simulink model "MIL_ASW"  (R2019b)
settings: Solver=FixedStepDiscrete  StartTime=0.0  StopTime=2  FixedStep=0.001  RelTol=1e-3  EnableMultiTasking=on
model workspace (MAT data in the model file):
  AccPedlCanVal : Simulink.Signal (value not decoded)
  AccPedlVal : Simulink.Signal (value not decoded)
  BrkPedlCanVal : Simulink.Signal (value not decoded)
  BrkPedlVal : Simulink.Signal (value not decoded)
  Cal1 : Simulink.Parameter (value not decoded)
  Cal10 : Simulink.Parameter (value not decoded)
  Cal11 : Simulink.Parameter (value not decoded)
  Cal12 : Simulink.Parameter (value not decoded)
  Cal2 : Simulink.Parameter (value not decoded)
  Cal3 : Simulink.Parameter (value not decoded)
  Cal4 : Simulink.Parameter (value not decoded)
  Cal5 : Simulink.Parameter (value not decoded)
  Cal6 : Simulink.Parameter (value not decoded)
  Cal7 : Simulink.Parameter (value not decoded)
  Cal8 : Simulink.Parameter (value not decoded)
  Cal9 : Simulink.Parameter (value not decoded)
  Clu1Act : Simulink.Signal (value not decoded)
  Clu1PTar : Simulink.Signal (value not decoded)
  Clu1Req : Simulink.Signal (value not decoded)
  Clu1TqTar : Simulink.Signal (value not decoded)
  Clu2Act : Simulink.Signal (value not decoded)
  Clu2PTar : Simulink.Signal (value not decoded)
  Clu2Req : Simulink.Signal (value not decoded)
  Clu2TqTar : Simulink.Signal (value not decoded)
  CluKissPtPLnch : Simulink.Parameter (value not decoded)
  CluOilTRawVal : Simulink.Signal (value not decoded)
  CluOilTVal : Simulink.Signal (value not decoded)
  CluOpenTqRatMax : Simulink.Parameter (value not decoded)
  CluPMap : Simulink.Parameter (value not decoded)
  CluPMax : Simulink.Parameter (value not decoded)
  CluPMaxGear1 : Simulink.Parameter (value not decoded)
  CluPMaxGear2 : Simulink.Parameter (value not decoded)
  CluPMaxGear3 : Simulink.Parameter (value not decoded)
  CluPMaxGear4 : Simulink.Parameter (value not decoded)
  CluPMaxGear5 : Simulink.Parameter (value not decoded)
  CluPMaxGear6 : Simulink.Parameter (value not decoded)
  CluPMaxGearR : Simulink.Parameter (value not decoded)
  CluPMin : Simulink.Parameter (value not decoded)
  CluPosnMax : Simulink.Parameter (value not decoded)
  CluSoln1IRawVal : Simulink.Signal (value not decoded)
  CluSoln1IReq : Simulink.Signal (value not decoded)
  CluSoln1IReqFlg : Simulink.Signal (value not decoded)
  CluSoln1IVal : Simulink.Signal (value not decoded)
  CluSoln1LineI : Simulink.Parameter (value not decoded)
  CluSoln1LineP : Simulink.Parameter (value not decoded)
  CluSoln1Pwm : Simulink.Signal (value not decoded)
  CluSoln2IRawVal : Simulink.Signal (value not decoded)
  CluSoln2IReq : Simulink.Signal (value not decoded)
  CluSoln2IReqFlg : Simulink.Signal (value not decoded)
  CluSoln2IVal : Simulink.Signal (value not decoded)
  CluSoln2LineI : Simulink.Parameter (value not decoded)
  CluSoln2LineP : Simulink.Parameter (value not decoded)
  CluSoln2Pwm : Simulink.Signal (value not decoded)
  CluTqMap : Simulink.Parameter (value not decoded)
  CrnkSpdRawVal : Simulink.Signal (value not decoded)
  CrnkSpdVal : Simulink.Signal (value not decoded)
  Drive_Intensity_Fuzzy : object (value not decoded)
  DrvIntenFzzy : Simulink.LookupTable (value not decoded)
  EngNIdle : Simulink.Parameter (value not decoded)
  EngNIdleMin : Simulink.Parameter (value not decoded)
  EngSpdCanVal : Simulink.Signal (value not decoded)
  EngThrCanVal : Simulink.Signal (value not decoded)
  EngTqAdd : Simulink.Parameter (value not decoded)
  EngTqCanVal : Simulink.Signal (value not decoded)
  EngTqIntvFlg : Simulink.Signal (value not decoded)
  EngTqIntvRat : Simulink.Signal (value not decoded)
  EngTqMapExtChartc : Simulink.Parameter (value not decoded)
  EngTqMapSpdIndx : Simulink.Parameter (value not decoded)
  EngTqMapThrtIndx : Simulink.Parameter (value not decoded)
  EngTqMapTqMax : Simulink.Parameter (value not decoded)
  EngTqMaxNorm : Simulink.Parameter (value not decoded)
  EngTqRef : Simulink.Parameter (value not decoded)
  EvenCluPRawVal : Simulink.Signal (value not decoded)
  EvenCluPVal : Simulink.Signal (value not decoded)
  EvenInpSpdRawVal : Simulink.Signal (value not decoded)
  EvenInpSpdVal : Simulink.Signal (value not decoded)
  FcnCallTime : Simulink.Parameter (value not decoded)
  FinalRat : Simulink.Parameter (value not decoded)
  Fork1A : Simulink.Parameter (value not decoded)
  Fork1Act : Simulink.Signal (value not decoded)
  Fork1B : Simulink.Parameter (value not decoded)
  Fork1DeltaSpdTar : Simulink.Parameter (value not decoded)
  Fork1MaxSpd1A : Simulink.Parameter (value not decoded)
  Fork1MaxSpd1B : Simulink.Parameter (value not decoded)
  Fork1MaxSpd2A : Simulink.Parameter (value not decoded)
  Fork1MaxSpd2B : Simulink.Parameter (value not decoded)
  Fork1PosnA : Simulink.Parameter (value not decoded)
  Fork1PosnB : Simulink.Parameter (value not decoded)
  Fork1PosnMaxSpd1A : Simulink.Parameter (value not decoded)
  Fork1PosnMaxSpd1B : Simulink.Parameter (value not decoded)
  Fork1PosnMaxSpd2A : Simulink.Parameter (value not decoded)
  Fork1PosnMaxSpd2B : Simulink.Parameter (value not decoded)
  Fork1PosnNeut : Simulink.Parameter (value not decoded)
  Fork1PosnNeutA : Simulink.Parameter (value not decoded)
  Fork1PosnNeutB : Simulink.Parameter (value not decoded)
  Fork1PosnRawVal : Simulink.Signal (value not decoded)
  Fork1PosnSyncA : Simulink.Parameter (value not decoded)
  Fork1PosnSyncB : Simulink.Parameter (value not decoded)
  Fork1PosnVal : Simulink.Signal (value not decoded)
  Fork1SyncTar : Simulink.Parameter (value not decoded)
  Fork2A : Simulink.Parameter (value not decoded)
  Fork2Act : Simulink.Signal (value not decoded)
  Fork2B : Simulink.Parameter (value not decoded)
  Fork2DeltaSpdTar : Simulink.Parameter (value not decoded)
  Fork2MaxSpd1A : Simulink.Parameter (value not decoded)
  Fork2MaxSpd1B : Simulink.Parameter (value not decoded)
  Fork2MaxSpd2A : Simulink.Parameter (value not decoded)
  Fork2MaxSpd2B : Simulink.Parameter (value not decoded)
  Fork2PosnA : Simulink.Parameter (value not decoded)
  Fork2PosnB : Simulink.Parameter (value not decoded)
  Fork2PosnMaxSpd1A : Simulink.Parameter (value not decoded)
  Fork2PosnMaxSpd1B : Simulink.Parameter (value not decoded)
  Fork2PosnMaxSpd2A : Simulink.Parameter (value not decoded)
  Fork2PosnMaxSpd2B : Simulink.Parameter (value not decoded)
  Fork2PosnNeut : Simulink.Parameter (value not decoded)
  Fork2PosnNeutA : Simulink.Parameter (value not decoded)
  Fork2PosnNeutB : Simulink.Parameter (value not decoded)
  Fork2PosnRawVal : Simulink.Signal (value not decoded)
  Fork2PosnSyncA : Simulink.Parameter (value not decoded)
  Fork2PosnSyncB : Simulink.Parameter (value not decoded)
  Fork2PosnVal : Simulink.Signal (value not decoded)
  Fork2SyncTar : Simulink.Parameter (value not decoded)
  Fork3A : Simulink.Parameter (value not decoded)
  Fork3Act : Simulink.Signal (value not decoded)
  Fork3B : Simulink.Parameter (value not decoded)
  Fork3DeltaSpdTar : Simulink.Parameter (value not decoded)
  Fork3MaxSpd1A : Simulink.Parameter (value not decoded)
  Fork3MaxSpd1B : Simulink.Parameter (value not decoded)
  Fork3MaxSpd2A : Simulink.Parameter (value not decoded)
  Fork3MaxSpd2B : Simulink.Parameter (value not decoded)
  Fork3PosnA : Simulink.Parameter (value not decoded)
  Fork3PosnB : Simulink.Parameter (value not decoded)
  Fork3PosnMaxSpd1A : Simulink.Parameter (value not decoded)
  Fork3PosnMaxSpd1B : Simulink.Parameter (value not decoded)
  Fork3PosnMaxSpd2A : Simulink.Parameter (value not decoded)
  Fork3PosnMaxSpd2B : Simulink.Parameter (value not decoded)
  Fork3PosnNeut : Simulink.Parameter (value not decoded)
  Fork3PosnNeutA : Simulink.Parameter (value not decoded)
  Fork3PosnNeutB : Simulink.Parameter (value not decoded)
  Fork3PosnRawVal : Simulink.Signal (value not decoded)
  Fork3PosnSyncA : Simulink.Parameter (value not decoded)
  Fork3PosnSyncB : Simulink.Parameter (value not decoded)
  Fork3PosnVal : Simulink.Signal (value not decoded)
  Fork3SyncTar : Simulink.Parameter (value not decoded)
  Fork4A : Simulink.Parameter (value not decoded)
  Fork4Act : Simulink.Signal (value not decoded)
  Fork4B : Simulink.Parameter (value not decoded)
  Fork4DeltaSpdTar : Simulink.Parameter (value not decoded)
  Fork4MaxSpd1A : Simulink.Parameter (value not decoded)
  Fork4MaxSpd1B : Simulink.Parameter (value not decoded)
  Fork4MaxSpd2A : Simulink.Parameter (value not decoded)
  Fork4MaxSpd2B : Simulink.Parameter (value not decoded)
  Fork4PosnA : Simulink.Parameter (value not decoded)
  Fork4PosnB : Simulink.Parameter (value not decoded)
  Fork4PosnMaxSpd1A : Simulink.Parameter (value not decoded)
  Fork4PosnMaxSpd1B : Simulink.Parameter (value not decoded)
  Fork4PosnMaxSpd2A : Simulink.Parameter (value not decoded)
  Fork4PosnMaxSpd2B : Simulink.Parameter (value not decoded)
  Fork4PosnNeut : Simulink.Parameter (value not decoded)
  Fork4PosnNeutA : Simulink.Parameter (value not decoded)
  Fork4PosnNeutB : Simulink.Parameter (value not decoded)
  Fork4PosnRawVal : Simulink.Signal (value not decoded)
  Fork4PosnSyncA : Simulink.Parameter (value not decoded)
  Fork4PosnSyncB : Simulink.Parameter (value not decoded)
  Fork4PosnVal : Simulink.Signal (value not decoded)
  Fork4SyncTar : Simulink.Parameter (value not decoded)
  FrntWhlRd : Simulink.Parameter (value not decoded)
  GearIdx : Simulink.Parameter (value not decoded)
  GearMax : Simulink.Parameter (value not decoded)
  GearRat : Simulink.Parameter (value not decoded)
  Launch_Engage_Fuzzy : object (value not decoded)
  LnchEngmtFzzy : Simulink.LookupTable (value not decoded)
  LubeSolnIRawVal : Simulink.Signal (value not decoded)
  LubeSolnIReq : Simulink.Signal (value not decoded)
  LubeSolnIVal : Simulink.Signal (value not decoded)
  LubeSolnLineI : Simulink.Parameter (value not decoded)
  LubeSolnLineP : Simulink.Parameter (value not decoded)
  LubeSolnPwm : Simulink.Signal (value not decoded)
  MaiLineSolnIRawVal : Simulink.Signal (value not decoded)
  MaiLineSolnIReq : Simulink.Signal (value not decoded)
  MaiLineSolnIVal : Simulink.Signal (value not decoded)
  MaiLineSolnLineI : Simulink.Parameter (value not decoded)
  MaiLineSolnLineP : Simulink.Parameter (value not decoded)
  MaiLineSolnPwm : Simulink.Signal (value not decoded)
  OddCluPRawVal : Simulink.Signal (value not decoded)
  OddCluPVal : Simulink.Signal (value not decoded)
  OddInpSpdRawVal : Simulink.Signal (value not decoded)
  OddInpSpdVal : Simulink.Signal (value not decoded)
  OutpSpdRawVal : Simulink.Signal (value not decoded)
  OutpSpdVal : Simulink.Signal (value not decoded)
  PsnsrLineP : Simulink.Parameter (value not decoded)
  PsnsrLineV : Simulink.Parameter (value not decoded)
  SftLvrCanVal : Simulink.Signal (value not decoded)
  SftLvrCfm : Simulink.Signal (value not decoded)
  SftLvrVal : Simulink.Signal (value not decoded)
  Shaft1GearAct : Simulink.Signal (value not decoded)
  Shaft1GearReq : Simulink.Signal (value not decoded)
  Shaft2GearAct : Simulink.Signal (value not decoded)
  Shaft2GearReq : Simulink.Signal (value not decoded)
  ShiftMux1SwtReq : Simulink.Signal (value not decoded)
  ShiftMux2SwtReq : Simulink.Signal (value not decoded)
  ShiftSdlEcoDwnSeln : Simulink.Parameter (value not decoded)
  ShiftSdlEcoDwnShift : Simulink.Parameter (value not decoded)
  ShiftSdlEcoUpSeln : Simulink.Parameter (value not decoded)
  ShiftSdlEcoUpShift : Simulink.Parameter (value not decoded)
  ShiftSdlPwrDwnSeln : Simulink.Parameter (value not decoded)
  ShiftSdlPwrDwnShift : Simulink.Parameter (value not decoded)
  ShiftSdlPwrUpSeln : Simulink.Parameter (value not decoded)
  ShiftSdlPwrUpShift : Simulink.Parameter (value not decoded)
  ShiftSdlSACDwnSeln : Simulink.Parameter (value not decoded)
  ShiftSdlSACDwnShift : Simulink.Parameter (value not decoded)
  ShiftSdlSACUpSeln : Simulink.Parameter (value not decoded)
  ShiftSdlSACUpShift : Simulink.Parameter (value not decoded)
  ShiftSdlThrPedlIdx : Simulink.Parameter (value not decoded)
  ShiftSoln1IRawVal : Simulink.Signal (value not decoded)
  ShiftSoln1IReq : Simulink.Signal (value not decoded)
  ShiftSoln1IVal : Simulink.Signal (value not decoded)
  ShiftSoln1LineI : Simulink.Parameter (value not decoded)
  ShiftSoln1LineP : Simulink.Parameter (value not decoded)
  ShiftSoln1Pwm : Simulink.Signal (value not decoded)
  ShiftSoln2IRawVal : Simulink.Signal (value not decoded)
  ShiftSoln2IReq : Simulink.Signal (value not decoded)
  ShiftSoln2IVal : Simulink.Signal (value not decoded)
  ShiftSoln2LineI : Simulink.Parameter (value not decoded)
  ShiftSoln2LineP : Simulink.Parameter (value not decoded)
  ShiftSoln2Pwm : Simulink.Signal (value not decoded)
  SolnOutpTRawVal : Simulink.Signal (value not decoded)
  SolnOutpTVal : Simulink.Signal (value not decoded)
  TSnsr1LineR : Simulink.Parameter (value not decoded)
  TSnsr2LineR : Simulink.Parameter (value not decoded)
  TrsmNrGearAct : Simulink.Signal (value not decoded)
  TrsmNrGearReq : Simulink.Signal (value not decoded)
  TrsmNrPreGearAct : Simulink.Signal (value not decoded)
  TrsmNrPreGearReq : Simulink.Signal (value not decoded)
  Tsnsr1LineT : Simulink.Parameter (value not decoded)
  Tsnsr2LineT : Simulink.Parameter (value not decoded)
  VehSpdCanVal : Simulink.Signal (value not decoded)
  VehSpdTrsmEstimd : Simulink.Signal (value not decoded)
  VehSpdVal : Simulink.Signal (value not decoded)
  VlvBodyTRawVal : Simulink.Signal (value not decoded)
  VlvBodyTVal : Simulink.Signal (value not decoded)
symbols that are objects in the model workspace (value not decoded): CluPMap, CluSoln1LineI, CluSoln1LineP, CluSoln2LineI, CluSoln2LineP, CluTqMap, EngNIdle, EngNIdleMin, EngTqMapThrtIndx, EngTqMapTqMax, EngTqMaxNorm, FcnCallTime, FinalRat, Fork1A, Fork1B, Fork1DeltaSpdTar, Fork1PosnA, Fork1PosnB, Fork1PosnMaxSpd1A, Fork1PosnMaxSpd1B, Fork1PosnMaxSpd2A, Fork1PosnMaxSpd2B, Fork1PosnNeut, Fork1PosnNeutA, Fork1PosnNeutB, Fork1PosnSyncA, Fork1PosnSyncB, Fork1SyncTar, Fork2A, Fork2B, Fork2DeltaSpdTar, Fork2PosnA, Fork2PosnB, Fork2PosnMaxSpd1A, Fork2PosnMaxSpd1B, Fork2PosnMaxSpd2A, Fork2PosnMaxSpd2B, Fork2PosnNeut, Fork2PosnNeutA, Fork2PosnNeutB, Fork2PosnSyncA, Fork2PosnSyncB, Fork2SyncTar, Fork3A, Fork3B, Fork3DeltaSpdTar, Fork3PosnA, Fork3PosnB, Fork3PosnMaxSpd1A, Fork3PosnMaxSpd1B, Fork3PosnMaxSpd2A, Fork3PosnMaxSpd2B, Fork3PosnNeut, Fork3PosnNeutA, Fork3PosnNeutB, Fork3PosnSyncA, Fork3PosnSyncB, Fork3SyncTar, Fork4A, Fork4B
undefined symbols (not defined in the file or in its folder): in1, out1
libraries: simulink x44, fuzblock x3
(part 4 of 10)

== system MIL_ASW/Application_Software_SHAW/ASW_ClutchControl_new/Clutch_Control_Strategy/Launch_Torque_Target ==
  EngThr : Inport  OutDataTypeStr=uint8  PortDimensions=1
  f : TriggerPort  TriggerType=function-call  VariantControl=(inherit)
      settings: CopyFcn=Stateflow.SLINSF.SimulinkMan.removeBlockPreDeleteFcn  PreDeleteFcn=Stateflow.SLINSF.SimulinkMan.unsafePredeleteFcn
  1-D Lookup Table : Lookup_n-D  NumberOfTableDimensions=1  BreakpointsForDimension1=EngTqMapThrtIndx  BreakpointsForDimension1DataTypeStr=Inherit: Inherit from 'Breakpoint data'  Table=EngTqMapTqMax  TableDataTypeStr=Inherit: Inherit from 'Table data'  ExtrapMethod=Clip  UseLastTableValue=on  OutDataTypeStr=Inherit: Inherit from 'Table data'  RndMeth=Simplest  InputSameDT=on
  Gain : Gain  Gain=6/5  OutDataTypeStr=uint16
  Tq : Outport  OutDataTypeStr=uint16  PortDimensions=1  VectorParamsAs1DForOutWhenUnconnected=off
  wires:
  1-D Lookup Table/1 -> Gain/1
  EngThr/1 -> 1-D Lookup Table/1
  Gain/1 -> Tq/1

== system MIL_ASW/Application_Software_SHAW/ASW_ClutchPressureControl/PID ==
  In1 : Inport
  1/100 : Gain  Gain=1/100  OutDataTypeStr=uint16
  1/1000ms : Gain  Gain=1/1000  OutDataTypeStr=int32
  Add1 : Sum  Inputs=+-+  OutDataTypeStr=int16
  Add7 : Sum  Inputs=+-  OutDataTypeStr=int16
  Add8 : Sum  Inputs=+++  OutDataTypeStr=int32
  Add9 : Sum  OutDataTypeStr=int32
  Gain2 : Gain  Gain=1000/FcnCallTime  OutDataTypeStr=int32
  Gain3 : Gain  Gain=FcnCallTime  OutDataTypeStr=int32
  Gain4 : Gain  Gain=1000  OutDataTypeStr=int32
  Gain6 : Gain  Gain=2  OutDataTypeStr=int32
  Kd*100 : Gain  Gain=0  OutDataTypeStr=int32
  Ki*100 : Gain  Gain=100  OutDataTypeStr=int32
  Kp*100 : Gain  Gain=15  OutDataTypeStr=int32
  Memory{1..3,5} (4 alike) : Memory  InheritSampleTime=on
  Saturation1 : Saturate  UpperLimit=100000  LowerLimit=0  OutDataTypeStr=int32
  Saturation2 : Saturate  UpperLimit=30000  LowerLimit=-30000
  Out1 : Outport  VectorParamsAs1DForOutWhenUnconnected=off
  wires:
  Add7/1 -> Kp*100/1
  Saturation2/1 -> Add9/2
  Ki*100/1 -> Gain3/1
  Kp*100/1 -> Gain4/1
  Memory2/1 -> Add7/2
  Saturation1/1 -> 1/100/1, Memory3/1
  Add9/1 -> Saturation1/1
  Add8/1 -> 1/1000ms/1
  In1/1 -> Add7/1, Memory1/1, Add1/1, Ki*100/1, Memory2/1
  Gain3/1 -> Add8/2
  Gain4/1 -> Add8/1
  Memory3/1 -> Add9/1
  Add1/1 -> Kd*100/1
  Gain6/1 -> Add1/2
  Kd*100/1 -> Gain2/1
  Memory5/1 -> Add1/3
  Gain2/1 -> Add8/3
  Memory1/1 -> Memory5/1, Gain6/1
  1/1000ms/1 -> Saturation2/1
  1/100/1 -> Out1/1

== system MIL_ASW/Application_Software_SHAW/ASW_ClutchPressureControl/PID1 ==
  In1 : Inport
  1/100 : Gain  Gain=1/100  OutDataTypeStr=uint16
  1/1000ms : Gain  Gain=1/1000  OutDataTypeStr=int32
  Add1 : Sum  Inputs=+-+  OutDataTypeStr=int16
  Add7 : Sum  Inputs=+-  OutDataTypeStr=int16
  Add8 : Sum  Inputs=+++  OutDataTypeStr=int32
  Add9 : Sum  OutDataTypeStr=int32
  Gain2 : Gain  Gain=1000/FcnCallTime  OutDataTypeStr=int32
  Gain3 : Gain  Gain=FcnCallTime  OutDataTypeStr=int32
  Gain4 : Gain  Gain=1000  OutDataTypeStr=int32
  Gain6 : Gain  Gain=2  OutDataTypeStr=int32
  Kd*100 : Gain  Gain=0  OutDataTypeStr=int32
  Ki*100 : Gain  Gain=100  OutDataTypeStr=int32
  Kp*100 : Gain  Gain=15  OutDataTypeStr=int32
  Memory{1..3,5} (4 alike) : Memory  InheritSampleTime=on
  Saturation1 : Saturate  UpperLimit=100000  LowerLimit=0  OutDataTypeStr=int32
  Saturation2 : Saturate  UpperLimit=30000  LowerLimit=-30000
  Out1 : Outport  VectorParamsAs1DForOutWhenUnconnected=off
  wires:
  Add7/1 -> Kp*100/1
  Saturation2/1 -> Add9/2
  Ki*100/1 -> Gain3/1
  Kp*100/1 -> Gain4/1
  Memory2/1 -> Add7/2
  Saturation1/1 -> 1/100/1, Memory3/1
  Add9/1 -> Saturation1/1
  Add8/1 -> 1/1000ms/1
  In1/1 -> Add7/1, Memory1/1, Add1/1, Ki*100/1, Memory2/1
  Gain3/1 -> Add8/2
  Gain4/1 -> Add8/1
  Memory3/1 -> Add9/1
  Add1/1 -> Kd*100/1
  Gain6/1 -> Add1/2
  Kd*100/1 -> Gain2/1
  Memory5/1 -> Add1/3
  Gain2/1 -> Add8/3
  Memory1/1 -> Memory5/1, Gain6/1
  1/1000ms/1 -> Saturation2/1
  1/100/1 -> Out1/1

== system MIL_ASW/Application_Software_SHAW/ASW_DrivingStrategy/Auto_Mode_Decision ==
  SftLvrVal : Inport
  AccPedlVal : Inport  Port=2
  BrkVal : Inport  Port=3
  BrkSig : Inport  Port=4
  VehSpdVal : Inport  Port=5
  CrnkSpdVal : Inport  Port=6
  TrsmNrGearAct : Inport  Port=7
  TrsmNrPreGearAct : Inport  Port=8
  DrvrInten : Inport  Port=9
  Bus Creator : BusCreator  Inputs=8
  Bus Selector : BusSelector  OutputSignals=AccPedlVal,TrsmNrPreGearAct,TrsmNrGearAct
  Bus Selector1 : BusSelector  OutputSignals=AccPedlVal,TrsmNrPreGearAct,TrsmNrGearAct
  Bus Selector2 : BusSelector  OutputSignals=AccPedlVal,TrsmNrPreGearAct,TrsmNrGearAct
  Bus Selector4 : BusSelector  OutputSignals=SftLvrVal,BrkPedlVal,BrkSig,CrnkSpdVal,TrsmNrGearAct,TrsmNrPreGearAct,VehSpdVal
  Bus Selector5 : BusSelector  OutputSignals=AccPedlVal,SftLvrVal,BrkPedlVal,BrkSig,CrnkSpdVal,TrsmNrGearAct,TrsmNrPreGearAct,VehSpdVal
  Demux : Demux
  EcoMod : Subsystem
  Eco_Spt_Schedule_Mix : Subsystem
  Mux : Mux
  Mux1 : Mux
  Mux2 : Mux
  SAC_Original : Subsystem
  SptMod : Subsystem
  TrsmNrGearTarCalcnAutMod : Stateflow chart  TreatAsAtomicUnit=on
  TrsmNrPreGearTarCalcnAutMod : Stateflow chart  TreatAsAtomicUnit=on
  TrsmNrPreGearTarAutMod : Outport  VectorParamsAs1DForOutWhenUnconnected=off
  TrsmNrGearTarAutMod : Outport  Port=2  VectorParamsAs1DForOutWhenUnconnected=off
  wires:
  Bus Selector/3 -> EcoMod/3(TrsmNrGearAct)  "<TrsmNrGearAct>"
  Bus Selector/1 -> EcoMod/1(AccPedlVal)  "<AccPedlVal>"
  SftLvrVal/1 -> Bus Creator/1
  AccPedlVal/1 -> Bus Creator/2
  BrkVal/1 -> Bus Creator/3
  VehSpdVal/1 -> Bus Creator/5
  CrnkSpdVal/1 -> Bus Creator/6
  TrsmNrGearAct/1 -> Bus Creator/7
  TrsmNrPreGearAct/1 -> Bus Creator/8
  EcoMod/1(UpSeln) -> Mux/1  "VehSpdUpSeln"
  EcoMod/2(DwnSeln) -> Mux/2  "VehSpdDwnSeln"
  Bus Selector4/1 -> TrsmNrPreGearTarCalcnAutMod/1(ShiftLvrVal)  "<SftLvrVal>"
  Bus Selector4/2 -> TrsmNrPreGearTarCalcnAutMod/2(BrkVal)  "<BrkPedlVal>"
  Bus Selector4/4 -> TrsmNrPreGearTarCalcnAutMod/4(EngN)  "<CrnkSpdVal>"
  Bus Selector4/5 -> TrsmNrPreGearTarCalcnAutMod/5(TrsmNrGearAct)  "<TrsmNrGearAct>"
  Bus Selector4/6 -> TrsmNrPreGearTarCalcnAutMod/6(TrsmNrPreGearAct)  "<TrsmNrPreGearAct>"
  Bus Selector4/7 -> TrsmNrPreGearTarCalcnAutMod/7(VehSpd)  "<VehSpdVal>"
  Bus Selector5/2 -> TrsmNrGearTarCalcnAutMod/2(ShiftLvrVal)  "<SftLvrVal>"
  Bus Selector5/3 -> TrsmNrGearTarCalcnAutMod/3(BrkVal)  "<BrkPedlVal>"
  Bus Selector5/5 -> TrsmNrGearTarCalcnAutMod/5(EngN)  "<CrnkSpdVal>"
  Bus Selector5/6 -> TrsmNrGearTarCalcnAutMod/6(TrsmNrGearAct)  "<TrsmNrGearAct>"
  Bus Selector5/7 -> TrsmNrGearTarCalcnAutMod/7(TrsmNrPreGearAct)  "<TrsmNrPreGearAct>"
  Bus Selector5/8 -> TrsmNrGearTarCalcnAutMod/8(VehSpd)  "<VehSpdVal>"
  EcoMod/3(UpShift) -> Mux/3  "VehSpdUpShift"
  EcoMod/4(DwnShift) -> Mux/4  "VehSpdDwnShift"
  TrsmNrGearTarCalcnAutMod/1(TrsmNrGearTarAutMod) -> TrsmNrGearTarAutMod/1  "TrsmNrGearTarAutMod"
  TrsmNrPreGearTarCalcnAutMod/1(TrsmNrPreGearTarAutMod) -> TrsmNrPreGearTarAutMod/1  "TrsmNrPreGearTarAutMod"
  BrkSig/1 -> Bus Creator/4
  Bus Selector4/3 -> TrsmNrPreGearTarCalcnAutMod/3(BrkSig)  "<BrkSig>"
  Bus Selector5/4 -> TrsmNrGearTarCalcnAutMod/4(BrkSig)  "<BrkSig>"
  Bus Selector/2 -> EcoMod/2(TrsmPreNrGearAct)  "<TrsmNrPreGearAct>"
  Bus Selector1/3 -> SptMod/3(TrsmNrGearAct)  "<TrsmNrGearAct>"
  Bus Selector1/1 -> SptMod/1(AccPedlVal)  "<AccPedlVal>"
  Bus Selector1/2 -> SptMod/2(TrsmPreNrGearAct)  "<TrsmNrPreGearAct>"
  Bus Selector2/2 -> SAC_Original/2(TrsmPreNrGearAct)  "<TrsmNrPreGearAct>"
  Bus Selector2/1 -> SAC_Original/1(AccPedlVal)  "<AccPedlVal>"
  Bus Selector2/3 -> SAC_Original/3(TrsmNrGearAct)  "<TrsmNrGearAct>"
  Bus Creator/1 -> Bus Selector1/1, Bus Selector2/1, Bus Selector/1, Bus Selector4/1, Bus Selector5/1
  Bus Selector5/1 -> TrsmNrGearTarCalcnAutMod/1(AccPedl)  "<AccPedlVal>"
  Demux/1 -> TrsmNrPreGearTarCalcnAutMod/8(VehSpdUpSeln)
  Demux/2 -> TrsmNrPreGearTarCalcnAutMod/9(VehSpdDwnSeln)
  Demux/3 -> TrsmNrGearTarCalcnAutMod/9(VehSpdUpShift)
  Demux/4 -> TrsmNrGearTarCalcnAutMod/10(VehSpdDwnShift)
  SptMod/4(DwnShift) -> Mux1/4  "VehSpdDwnShift"
  SptMod/3(UpShift) -> Mux1/3  "VehSpdUpShift"
  SptMod/2(DwnSeln) -> Mux1/2  "VehSpdDwnSeln"
  SptMod/1(UpSeln) -> Mux1/1  "VehSpdUpSeln"
  SAC_Original/1(UpSeln) -> Mux2/1  "VehSpdUpSeln"
  SAC_Original/2(DwnSeln) -> Mux2/2  "VehSpdDwnSeln"
  SAC_Original/3(UpShift) -> Mux2/3  "VehSpdUpShift"
  SAC_Original/4(DwnShift) -> Mux2/4  "VehSpdDwnShift"
  DrvrInten/1 -> Eco_Spt_Schedule_Mix/1(DrvrInten)
  Mux1/1 -> Eco_Spt_Schedule_Mix/3(SptShiftSpd)
  Mux/1 -> Eco_Spt_Schedule_Mix/2(EcoShiftSpd)
  Eco_Spt_Schedule_Mix/1(MixShiftSpd) -> Demux/1

== system MIL_ASW/Application_Software_SHAW/ASW_DrivingStrategy/Driver_Detection ==
  AccPedl : Inport  OutDataTypeStr=uint8  PortDimensions=1
  Constant1 : Constant  Value=100  OutDataTypeStr=int16
  Constant2 : Constant  Value=FcnCallTime  OutDataTypeStr=uint8
  Constant3 : Constant  Value=1000  OutDataTypeStr=int16
  Divide : Product  Inputs=*/  OutDataTypeStr=int16
  Divide1 : Product  Inputs=*/  OutDataTypeStr=int16
  Fuzzy Logic Controller : fuzblock/Fuzzy Logic  Controller  Commented=on  FIS='Drive_Intention_Fuzzy.fis'  OutputSampleNumber=101  DataType=single  FuzzifiedInputs=off  RuleFiringStrengths=off  RuleOutputs=off  AggregatedOutputs=off  SimulateUsing=Interpreted execution  OutOfRangeInputValueMessage=warning  NoRuleFiredMessage=warning  EmptyOutputFuzzySetMessage=warning
  Mux : Mux  Commented=on  Inputs=2
  Product : Product  OutDataTypeStr=int16
  Saturation : Saturate  UpperLimit=100  LowerLimit=0  OutDataTypeStr=int16
  Saturation1 : Saturate  UpperLimit=300  LowerLimit=-300  OutDataTypeStr=int16
  Saturation2 : Saturate  UpperLimit=100  LowerLimit=0  OutDataTypeStr=int16
  Scope1 : Scope
  Scope2 : Scope
  Scope3 : Scope
  Subtract1 : Sum  Inputs=+-  OutDataTypeStr=int16
  Variable Integer Delay : Delay  DelayLengthSource=Input port
      settings: InputPortMap=u0,p1
  fuzzy_lookup_table : Lookup_n-D  DataSpecification=Lookup table object  LookupTableObject=DrvIntenFzzy  BreakpointsForDimension1=in1  BreakpointsForDimension2=in1  BreakpointsForDimension1DataTypeStr=int16  BreakpointsForDimension2DataTypeStr=int16  Table=out1  TableDataTypeStr=int16  ExtrapMethod=Clip  UseLastTableValue=on  InternalRulePriority=Speed  OutDataTypeStr=Inherit: Inherit from 'Table data'  RndMeth=Simplest  InputSameDT=on
  Inten : Outport  VectorParamsAs1DForOutWhenUnconnected=off
  wires:
  Divide1/1 -> Product/2
  Divide/1 -> Variable Integer Delay/2
  Constant1/1 -> Divide1/2, Divide/1
  Subtract1/1 -> Product/1
  Saturation2/1 -> Inten/1, Scope1/1
  Constant2/1 -> Divide/2
  Variable Integer Delay/1 -> Subtract1/2
  fuzzy_lookup_table/1 -> Saturation2/1
  Saturation1/1 -> Scope2/1, fuzzy_lookup_table/2, Mux/2
  Saturation/1 -> Mux/1, Scope3/1, fuzzy_lookup_table/1
  Constant3/1 -> Divide1/1
  AccPedl/1 -> Saturation/1, Variable Integer Delay/1, Subtract1/1
  Product/1 -> Saturation1/1
  Mux/1 -> Fuzzy Logic Controller/1

== system MIL_ASW/Application_Software_SHAW/ASW_DrivingStrategy/Fast_Off_Detection ==
  In1 : Inport
  Out1 : Outport  VectorParamsAs1DForOutWhenUnconnected=off
  wires:
  In1/1 -> Out1/1

== system MIL_ASW/Application_Software_SHAW/ASW_DrivingStrategy/Load_Detection ==
  In1 : Inport
  Out1 : Outport  VectorParamsAs1DForOutWhenUnconnected=off
  wires:
  In1/1 -> Out1/1

== system MIL_ASW/Application_Software_SHAW/ASW_DrivingStrategy/Manual_Mode_Decision ==
  In1 : Inport
  Out1 : Outport  VectorParamsAs1DForOutWhenUnconnected=off
  wires:
  In1/1 -> Out1/1

== system MIL_ASW/Application_Software_SHAW/ASW_DrivingStrategy/Road_Detection ==
  In1 : Inport
  Out1 : Outport  VectorParamsAs1DForOutWhenUnconnected=off
  wires:
  In1/1 -> Out1/1

== system MIL_ASW/Application_Software_SHAW/ASW_DrivingStrategy/Synthesis_Check ==
  SftLvrVal : Inport
  TrsmNrPreGearTarAutMod : Inport  Port=2
  TrsmNrGearTarAutMod : Inport  Port=3
  Compare To Constant : simulink/Logic and Bit Operations/Compare To Constant  relop===  const=0  OutDataTypeStr=uint8
  Compare To Constant2 : simulink/Logic and Bit Operations/Compare To Constant  relop===  const=2  OutDataTypeStr=uint8
  Constant : Constant  Value=0  OutDataTypeStr=uint8
  Logical Operator : Logic  Operator=OR  AllPortsSameDT=off
  Switch : Switch  Criteria=u2 ~= 0  OutDataTypeStr=uint8
  Switch1 : Switch  Criteria=u2 ~= 0  OutDataTypeStr=uint8
  TrsmNrPreGearReq : Outport  VectorParamsAs1DForOutWhenUnconnected=off
  TrsmNrGearReq : Outport  Port=2  VectorParamsAs1DForOutWhenUnconnected=off
  wires:
  SftLvrVal/1 -> Compare To Constant2/1, Compare To Constant/1
  Compare To Constant/1 -> Logical Operator/1
  Compare To Constant2/1 -> Logical Operator/2
  Logical Operator/1 -> Switch1/2, Switch/2
  TrsmNrPreGearTarAutMod/1 -> Switch/3
  Switch/1 -> TrsmNrPreGearReq/1
  Constant/1 -> Switch1/1, Switch/1
  TrsmNrGearTarAutMod/1 -> Switch1/3
  Switch1/1 -> TrsmNrGearReq/1

== system MIL_ASW/Application_Software_SHAW/ASW_GearPositioner/Fork1/Ini_ForkAct ==
  PosnAct : Inport  OutDataTypeStr=uint16
  f : TriggerPort  TriggerType=function-call  VariantControl=(inherit)
      settings: CopyFcn=Stateflow.SLINSF.SimulinkMan.removeBlockPreDeleteFcn  PreDeleteFcn=Stateflow.SLINSF.SimulinkMan.unsafePredeleteFcn
  Constant10 : Constant  Value=Fork1A  OutDataTypeStr=uint8
  Constant11 : Constant  Value=Fork1A  OutDataTypeStr=uint8
  Constant12 : Constant  Value=Fork1B  OutDataTypeStr=uint8
  Constant13 : Constant  Value=Fork1B  OutDataTypeStr=uint8
  Constant5 : Constant  Value=Fork1PosnNeutA  OutDataTypeStr=uint16
  Constant6 : Constant  Value=Fork1PosnSyncA  OutDataTypeStr=uint16
  Constant7 : Constant  Value=Fork1PosnNeutB  OutDataTypeStr=uint16
  Constant8 : Constant  Value=Fork1PosnSyncB  OutDataTypeStr=uint16
  Constant9 : Constant  Value=0  OutDataTypeStr=uint8
  Gain : Gain  Gain=10  OutDataTypeStr=Inherit: Same as input
  Gain1 : Gain  Gain=10  OutDataTypeStr=Inherit: Same as input
  If : If  NumInputs=5  IfExpression=u1<=u3&u1>=u4  ElseIfExpressions=u1>u2, u1<=u2&u1>u3, u1<u4&u1>=u5, u1<u5  ShowElse=off
  Merge : Merge  Inputs=5
  position_A : Subsystem  TreatAsAtomicUnit=on
  position_B : Subsystem  TreatAsAtomicUnit=on
  position_between_Neutral_A : Subsystem  TreatAsAtomicUnit=on
  position_between_Neutral_B : Subsystem  TreatAsAtomicUnit=on
  position_neutral : Subsystem  TreatAsAtomicUnit=on
  ForkAct : Outport  VectorParamsAs1DForOutWhenUnconnected=off
  wires:
  PosnAct/1 -> If/1
  Constant5/1 -> If/3
  Constant6/1 -> If/2
  Constant7/1 -> If/4
  Constant8/1 -> If/5
  Constant9/1 -> position_neutral/1(In1)
  If/1 -> position_neutral/Action
  Constant10/1 -> position_A/1(In1)
  If/2 -> position_A/Action
  If/3 -> position_between_Neutral_A/Action
  Constant11/1 -> Gain/1
  Gain/1 -> position_between_Neutral_A/1(In1)
  Constant12/1 -> Gain1/1
  Gain1/1 -> position_between_Neutral_B/1(In1)
  If/4 -> position_between_Neutral_B/Action
  Constant13/1 -> position_B/1(In1)
  If/5 -> position_B/Action
  position_between_Neutral_A/1(Out1) -> Merge/3
  position_between_Neutral_B/1(Out1) -> Merge/4
  position_A/1(Out1) -> Merge/2
  position_B/1(Out1) -> Merge/5
  position_neutral/1(Out1) -> Merge/1
  Merge/1 -> ForkAct/1

== system MIL_ASW/Application_Software_SHAW/ASW_GearPositioner/Fork1/PosnTar ==
  PosnAct : Inport  OutDataTypeStr=uint16
  f : TriggerPort  TriggerType=function-call  VariantControl=(inherit)
      settings: CopyFcn=Stateflow.SLINSF.SimulinkMan.removeBlockPreDeleteFcn  PreDeleteFcn=Stateflow.SLINSF.SimulinkMan.unsafePredeleteFcn
  Constant : Constant  Value=1000  OutDataTypeStr=uint16
  Constant1 : Constant  Value=FcnCallTime  OutDataTypeStr=uint8
  Divide : Product  Inputs=*/  OutDataTypeStr=uint16
  Fork1 Position Lookup Table : Lookup_n-D  NumberOfTableDimensions=1  BreakpointsForDimension1=[Fork1PosnB,Fork1PosnMaxSpd2B,Fork1PosnSyncB,Fork1PosnMaxSpd1B,Fork1PosnNeut,Fork1PosnMaxSpd1A,Fork1PosnSyncA,Fork1PosnMaxSpd2A,Fork1PosnA]  BreakpointsForDimension1DataTypeStr=Inherit: Inherit from 'Breakpoint data'  Table=uint16([1000,4000,4000,3000,3000,3000,4000,4000,1000])  TableDataTypeStr=Inherit: Inherit from 'Table data'  ExtrapMethod=Clip  OutDataTypeStr=Inherit: Inherit from 'Table data'  RndMeth=Simplest  InputSameDT=on
  Product : Product  OutDataTypeStr=uint32
  PosnTar : Outport  VectorParamsAs1DForOutWhenUnconnected=off
  wires:
  PosnAct/1 -> Fork1 Position Lookup Table/1
  Fork1 Position Lookup Table/1 -> Product/2
  Product/1 -> Divide/1
  Constant/1 -> Divide/2
  Divide/1 -> PosnTar/1
  Constant1/1 -> Product/1

== system MIL_ASW/Application_Software_SHAW/ASW_GearPositioner/Fork2/Ini_ForkAct ==
  PosnAct : Inport  OutDataTypeStr=uint16
  f : TriggerPort  TriggerType=function-call  VariantControl=(inherit)
      settings: CopyFcn=Stateflow.SLINSF.SimulinkMan.removeBlockPreDeleteFcn  PreDeleteFcn=Stateflow.SLINSF.SimulinkMan.unsafePredeleteFcn
  Constant10 : Constant  Value=Fork2A  OutDataTypeStr=uint8
  Constant11 : Constant  Value=Fork2A  OutDataTypeStr=uint8
  Constant12 : Constant  Value=Fork2B  OutDataTypeStr=uint8
  Constant13 : Constant  Value=Fork2B  OutDataTypeStr=uint8
  Constant5 : Constant  Value=Fork2PosnNeutA  OutDataTypeStr=uint16
  Constant6 : Constant  Value=Fork2PosnSyncA  OutDataTypeStr=uint16
  Constant7 : Constant  Value=Fork2PosnNeutB  OutDataTypeStr=uint16
  Constant8 : Constant  Value=Fork2PosnSyncB  OutDataTypeStr=uint16
  Constant9 : Constant  Value=0  OutDataTypeStr=uint8
  Gain : Gain  Gain=10  OutDataTypeStr=Inherit: Same as input
  Gain1 : Gain  Gain=10  OutDataTypeStr=Inherit: Same as input
  If : If  NumInputs=5  IfExpression=u1<=u3&u1>=u4  ElseIfExpressions=u1>u2, u1<=u2&u1>u3, u1<u4&u1>=u5, u1<u5  ShowElse=off
  Merge : Merge  Inputs=5
  position_A : Subsystem  TreatAsAtomicUnit=on
  position_B : Subsystem  TreatAsAtomicUnit=on
  position_between_Neutral_A : Subsystem  TreatAsAtomicUnit=on
  position_between_Neutral_B : Subsystem  TreatAsAtomicUnit=on
  position_neutral : Subsystem  TreatAsAtomicUnit=on
  ForkAct : Outport  VectorParamsAs1DForOutWhenUnconnected=off
  wires:
  PosnAct/1 -> If/1
  Constant5/1 -> If/3
  Constant6/1 -> If/2
  Constant7/1 -> If/4
  Constant8/1 -> If/5
  Constant9/1 -> position_neutral/1(In1)
  If/1 -> position_neutral/Action
  Constant10/1 -> position_A/1(In1)
  If/2 -> position_A/Action
  If/3 -> position_between_Neutral_A/Action
  Constant11/1 -> Gain/1
  Gain/1 -> position_between_Neutral_A/1(In1)
  Constant12/1 -> Gain1/1
  Gain1/1 -> position_between_Neutral_B/1(In1)
  If/4 -> position_between_Neutral_B/Action
  Constant13/1 -> position_B/1(In1)
  If/5 -> position_B/Action
  position_between_Neutral_A/1(Out1) -> Merge/3
  position_between_Neutral_B/1(Out1) -> Merge/4
  position_A/1(Out1) -> Merge/2
  position_B/1(Out1) -> Merge/5
  position_neutral/1(Out1) -> Merge/1
  Merge/1 -> ForkAct/1

== system MIL_ASW/Application_Software_SHAW/ASW_GearPositioner/Fork2/PosnTar ==
  PosnAct : Inport  OutDataTypeStr=uint16
  f : TriggerPort  TriggerType=function-call  VariantControl=(inherit)
      settings: CopyFcn=Stateflow.SLINSF.SimulinkMan.removeBlockPreDeleteFcn  PreDeleteFcn=Stateflow.SLINSF.SimulinkMan.unsafePredeleteFcn
  Constant : Constant  Value=1000  OutDataTypeStr=uint16
  Constant1 : Constant  Value=FcnCallTime  OutDataTypeStr=uint8
  Divide : Product  Inputs=*/  OutDataTypeStr=uint16
  Fork2 Position Lookup Table : Lookup_n-D  NumberOfTableDimensions=1  BreakpointsForDimension1=[Fork2PosnB,Fork2PosnMaxSpd2B,Fork2PosnSyncB,Fork2PosnMaxSpd1B,Fork2PosnNeut,Fork2PosnMaxSpd1A,Fork2PosnSyncA,Fork2PosnMaxSpd2A,Fork2PosnA]  BreakpointsForDimension1DataTypeStr=Inherit: Inherit from 'Breakpoint data'  Table=uint16([1000,4000,4000,3000,3000,3000,4000,4000,1000])  TableDataTypeStr=Inherit: Inherit from 'Table data'  ExtrapMethod=Clip  OutDataTypeStr=Inherit: Inherit from 'Table data'  RndMeth=Simplest  InputSameDT=on
  Product : Product  OutDataTypeStr=uint32
  PosnTar : Outport  VectorParamsAs1DForOutWhenUnconnected=off
  wires:
  PosnAct/1 -> Fork2 Position Lookup Table/1
  Fork2 Position Lookup Table/1 -> Product/2
  Product/1 -> Divide/1
  Constant/1 -> Divide/2
  Divide/1 -> PosnTar/1
  Constant1/1 -> Product/1

== system MIL_ASW/Application_Software_SHAW/ASW_GearPositioner/Fork3/Ini_ForkAct ==
  PosnAct : Inport  OutDataTypeStr=uint16
  f : TriggerPort  TriggerType=function-call  VariantControl=(inherit)
      settings: CopyFcn=Stateflow.SLINSF.SimulinkMan.removeBlockPreDeleteFcn  PreDeleteFcn=Stateflow.SLINSF.SimulinkMan.unsafePredeleteFcn
  Constant10 : Constant  Value=Fork3A  OutDataTypeStr=uint8
  Constant11 : Constant  Value=Fork3A  OutDataTypeStr=uint8
  Constant12 : Constant  Value=Fork3B  OutDataTypeStr=uint8
  Constant13 : Constant  Value=Fork3B  OutDataTypeStr=uint8
  Constant5 : Constant  Value=Fork3PosnNeutA  OutDataTypeStr=uint16
  Constant6 : Constant  Value=Fork3PosnSyncA  OutDataTypeStr=uint16
  Constant7 : Constant  Value=Fork3PosnNeutB  OutDataTypeStr=uint16
  Constant8 : Constant  Value=Fork3PosnSyncB  OutDataTypeStr=uint16
  Constant9 : Constant  Value=0  OutDataTypeStr=uint8
  Gain : Gain  Gain=10  OutDataTypeStr=Inherit: Same as input
  Gain1 : Gain  Gain=10  OutDataTypeStr=Inherit: Same as input
  If : If  NumInputs=5  IfExpression=u1<=u3&u1>=u4  ElseIfExpressions=u1>u2, u1<=u2&u1>u3, u1<u4&u1>=u5, u1<u5  ShowElse=off
  Merge : Merge  Inputs=5
  position_A : Subsystem  TreatAsAtomicUnit=on
  position_B : Subsystem  TreatAsAtomicUnit=on
  position_between_Neutral_A : Subsystem  TreatAsAtomicUnit=on
  position_between_Neutral_B : Subsystem  TreatAsAtomicUnit=on
  position_neutral : Subsystem  TreatAsAtomicUnit=on
  ForkAct : Outport  VectorParamsAs1DForOutWhenUnconnected=off
  wires:
  Merge/1 -> ForkAct/1
  position_neutral/1(Out1) -> Merge/1
  position_B/1(Out1) -> Merge/5
  position_A/1(Out1) -> Merge/2
  position_between_Neutral_B/1(Out1) -> Merge/4
  position_between_Neutral_A/1(Out1) -> Merge/3
  If/5 -> position_B/Action
  Constant13/1 -> position_B/1(In1)
  If/4 -> position_between_Neutral_B/Action
  Gain1/1 -> position_between_Neutral_B/1(In1)
  Constant12/1 -> Gain1/1
  Gain/1 -> position_between_Neutral_A/1(In1)
  Constant11/1 -> Gain/1
  If/3 -> position_between_Neutral_A/Action
  If/2 -> position_A/Action
  Constant10/1 -> position_A/1(In1)
  If/1 -> position_neutral/Action
  Constant9/1 -> position_neutral/1(In1)
  Constant8/1 -> If/5
  Constant7/1 -> If/4
  Constant6/1 -> If/2
  Constant5/1 -> If/3
  PosnAct/1 -> If/1

== system MIL_ASW/Application_Software_SHAW/ASW_GearPositioner/Fork3/PosnTar ==
  ForkAct : Inport  OutDataTypeStr=uint16
  f : TriggerPort  TriggerType=function-call  VariantControl=(inherit)
      settings: CopyFcn=Stateflow.SLINSF.SimulinkMan.removeBlockPreDeleteFcn  PreDeleteFcn=Stateflow.SLINSF.SimulinkMan.unsafePredeleteFcn
  Constant : Constant  Value=1000  OutDataTypeStr=uint16
  Constant1 : Constant  Value=FcnCallTime  OutDataTypeStr=uint8
  Divide : Product  Inputs=*/  OutDataTypeStr=uint16
  Fork3 Position Lookup Table : Lookup_n-D  NumberOfTableDimensions=1  BreakpointsForDimension1=[Fork3PosnB,Fork3PosnMaxSpd2B,Fork3PosnSyncB,Fork3PosnMaxSpd1B,Fork3PosnNeut,Fork3PosnMaxSpd1A,Fork3PosnSyncA,Fork3PosnMaxSpd2A,Fork3PosnA]  BreakpointsForDimension1DataTypeStr=Inherit: Inherit from 'Breakpoint data'  Table=uint16([1000,4000,4000,3000,3000,3000,4000,4000,1000])  TableDataTypeStr=Inherit: Inherit from 'Table data'  ExtrapMethod=Clip  OutDataTypeStr=Inherit: Inherit from 'Table data'  RndMeth=Simplest  InputSameDT=on
  Product : Product  OutDataTypeStr=uint32
  PosnTar : Outport  VectorParamsAs1DForOutWhenUnconnected=off
  wires:
  ForkAct/1 -> Fork3 Position Lookup Table/1
  Fork3 Position Lookup Table/1 -> Product/2
  Product/1 -> Divide/1
  Constant/1 -> Divide/2
  Divide/1 -> PosnTar/1
  Constant1/1 -> Product/1

== system MIL_ASW/Application_Software_SHAW/ASW_GearPositioner/Fork4/Ini_ForkAct ==
  PosnAct : Inport  OutDataTypeStr=uint16
  f : TriggerPort  TriggerType=function-call  VariantControl=(inherit)
      settings: CopyFcn=Stateflow.SLINSF.SimulinkMan.removeBlockPreDeleteFcn  PreDeleteFcn=Stateflow.SLINSF.SimulinkMan.unsafePredeleteFcn
  Constant10 : Constant  Value=Fork4A  OutDataTypeStr=uint8
  Constant11 : Constant  Value=Fork4A  OutDataTypeStr=uint8
  Constant12 : Constant  Value=Fork4B  OutDataTypeStr=uint8
  Constant13 : Constant  Value=Fork4B  OutDataTypeStr=uint8
  Constant5 : Constant  Value=Fork4PosnNeutA  OutDataTypeStr=uint16
  Constant6 : Constant  Value=Fork4PosnSyncA  OutDataTypeStr=uint16
  Constant7 : Constant  Value=Fork4PosnNeutB  OutDataTypeStr=uint16
  Constant8 : Constant  Value=Fork4PosnSyncB  OutDataTypeStr=uint16
  Constant9 : Constant  Value=0  OutDataTypeStr=uint8
  Gain : Gain  Gain=10  OutDataTypeStr=Inherit: Same as input
  Gain1 : Gain  Gain=10  OutDataTypeStr=Inherit: Same as input
  If : If  NumInputs=5  IfExpression=u1<=u3&u1>=u4  ElseIfExpressions=u1>u2, u1<=u2&u1>u3, u1<u4&u1>=u5, u1<u5  ShowElse=off
  Merge : Merge  Inputs=5
  position_A : Subsystem  TreatAsAtomicUnit=on
  position_B : Subsystem  TreatAsAtomicUnit=on
  position_between_Neutral_A : Subsystem  TreatAsAtomicUnit=on
  position_between_Neutral_B : Subsystem  TreatAsAtomicUnit=on
  position_neutral : Subsystem  TreatAsAtomicUnit=on
  ForkAct : Outport  VectorParamsAs1DForOutWhenUnconnected=off
  wires:
  PosnAct/1 -> If/1
  Constant5/1 -> If/3
  Constant6/1 -> If/2
  Constant7/1 -> If/4
  Constant8/1 -> If/5
  Constant9/1 -> position_neutral/1(In1)
  If/1 -> position_neutral/Action
  Constant10/1 -> position_A/1(In1)
  If/2 -> position_A/Action
  If/3 -> position_between_Neutral_A/Action
  Constant11/1 -> Gain/1
  Gain/1 -> position_between_Neutral_A/1(In1)
  Constant12/1 -> Gain1/1
  Gain1/1 -> position_between_Neutral_B/1(In1)
  If/4 -> position_between_Neutral_B/Action
  Constant13/1 -> position_B/1(In1)
  If/5 -> position_B/Action
  position_between_Neutral_A/1(Out1) -> Merge/3
  position_between_Neutral_B/1(Out1) -> Merge/4
  position_A/1(Out1) -> Merge/2
  position_B/1(Out1) -> Merge/5
  position_neutral/1(Out1) -> Merge/1
  Merge/1 -> ForkAct/1

== system MIL_ASW/Application_Software_SHAW/ASW_GearPositioner/Fork4/PosnTar ==
  ForkAct : Inport  OutDataTypeStr=uint16
  f : TriggerPort  TriggerType=function-call  VariantControl=(inherit)
      settings: CopyFcn=Stateflow.SLINSF.SimulinkMan.removeBlockPreDeleteFcn  PreDeleteFcn=Stateflow.SLINSF.SimulinkMan.unsafePredeleteFcn
  Constant : Constant  Value=1000  OutDataTypeStr=uint16
  Constant1 : Constant  Value=FcnCallTime  OutDataTypeStr=uint8
  Divide : Product  Inputs=*/  OutDataTypeStr=uint16
  Fork4 Position Lookup Table : Lookup_n-D  NumberOfTableDimensions=1  BreakpointsForDimension1=[Fork4PosnB,Fork4PosnMaxSpd2B,Fork4PosnSyncB,Fork4PosnMaxSpd1B,Fork4PosnNeut,Fork4PosnMaxSpd1A,Fork4PosnSyncA,Fork4PosnMaxSpd2A,Fork4PosnA]  BreakpointsForDimension1DataTypeStr=Inherit: Inherit from 'Breakpoint data'  Table=uint16([1000,4000,4000,3000,3000,3000,4000,4000,1000])  TableDataTypeStr=Inherit: Inherit from 'Table data'  ExtrapMethod=Clip  OutDataTypeStr=Inherit: Inherit from 'Table data'  RndMeth=Simplest  InputSameDT=on
  Product : Product  OutDataTypeStr=uint32
  PosnTar : Outport  VectorParamsAs1DForOutWhenUnconnected=off
  wires:
  ForkAct/1 -> Fork4 Position Lookup Table/1
  Fork4 Position Lookup Table/1 -> Product/2
  Product/1 -> Divide/1
  Constant/1 -> Divide/2
  Divide/1 -> PosnTar/1
  Constant1/1 -> Product/1

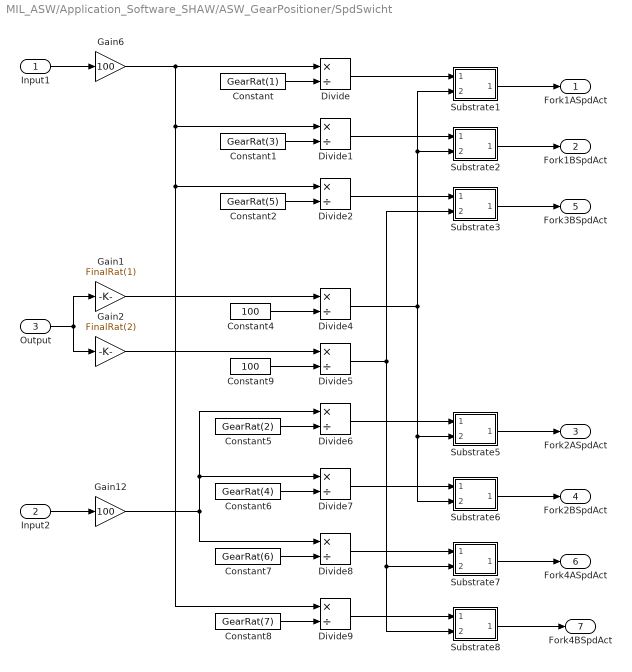
== system MIL_ASW/Application_Software_SHAW/ASW_GearPositioner/SpdSwicht ==
  Input1 : Inport
  Input2 : Inport  Port=2
  Output : Inport  Port=3
  Constant : Constant  Value=GearRat(1)  OutDataTypeStr=uint16
  Constant1 : Constant  Value=GearRat(3)  OutDataTypeStr=uint16
  Constant2 : Constant  Value=GearRat(5)  OutDataTypeStr=uint16
  Constant4 : Constant  Value=100  OutDataTypeStr=uint16
  Constant5 : Constant  Value=GearRat(2)  OutDataTypeStr=uint16
  Constant6 : Constant  Value=GearRat(4)  OutDataTypeStr=uint16
  Constant7 : Constant  Value=GearRat(6)  OutDataTypeStr=uint16
  Constant8 : Constant  Value=GearRat(7)  OutDataTypeStr=uint16
  Constant9 : Constant  Value=100  OutDataTypeStr=uint16
  Divide{,1..2,4..9} (9 alike) : Product  Inputs=*/  OutDataTypeStr=uint16
  Gain1 : Gain  Gain=FinalRat(1)  ParamDataTypeStr=uint16
  Gain12 : Gain  Gain=100
  Gain2 : Gain  Gain=FinalRat(2)  ParamDataTypeStr=uint16
  Gain6 : Gain  Gain=100
  Substrate1 : Subsystem
  Substrate2 : Subsystem
  Substrate3 : Subsystem
  Substrate5 : Subsystem
  Substrate6 : Subsystem
  Substrate7 : Subsystem
  Substrate8 : Subsystem
  Fork1ASpdAct : Outport  VectorParamsAs1DForOutWhenUnconnected=off
  Fork1BSpdAct : Outport  Port=2  VectorParamsAs1DForOutWhenUnconnected=off
  Fork2ASpdAct : Outport  Port=3  VectorParamsAs1DForOutWhenUnconnected=off
  Fork2BSpdAct : Outport  Port=4  VectorParamsAs1DForOutWhenUnconnected=off
  Fork3BSpdAct : Outport  Port=5  VectorParamsAs1DForOutWhenUnconnected=off
  Fork4ASpdAct : Outport  Port=6  VectorParamsAs1DForOutWhenUnconnected=off
  Fork4BSpdAct : Outport  Port=7  VectorParamsAs1DForOutWhenUnconnected=off
  wires:
  Divide4/1 -> Substrate6/2(In2), Substrate5/2(In2), Substrate2/2(In2), Substrate1/2(In2)
  Constant8/1 -> Divide9/2
  Constant7/1 -> Divide8/2
  Constant6/1 -> Divide7/2
  Constant5/1 -> Divide6/2
  Constant4/1 -> Divide4/2
  Constant2/1 -> Divide2/2
  Constant1/1 -> Divide1/2
  Constant/1 -> Divide/2
  Gain6/1 -> Divide9/1, Divide2/1, Divide1/1, Divide/1
  Input2/1 -> Gain12/1
  Substrate8/1(Out1) -> Fork4BSpdAct/1
  Substrate7/1(Out1) -> Fork4ASpdAct/1
  Divide9/1 -> Substrate8/1(In1)
  Divide8/1 -> Substrate7/1(In1)
  Substrate6/1(Out1) -> Fork2BSpdAct/1
  Divide7/1 -> Substrate6/1(In1)
  Substrate5/1(Out1) -> Fork2ASpdAct/1
  Divide6/1 -> Substrate5/1(In1)
  Substrate3/1(Out1) -> Fork3BSpdAct/1
  Divide2/1 -> Substrate3/1(In1)
  Substrate2/1(Out1) -> Fork1BSpdAct/1
  Divide1/1 -> Substrate2/1(In1)
  Substrate1/1(Out1) -> Fork1ASpdAct/1
  Output/1 -> Gain1/1, Gain2/1
  Divide/1 -> Substrate1/1(In1)
  Input1/1 -> Gain6/1
  Constant9/1 -> Divide5/2
  Gain1/1 -> Divide4/1
  Gain2/1 -> Divide5/1
  Gain12/1 -> Divide8/1, Divide7/1, Divide6/1
  Divide5/1 -> Substrate3/2(In2), Substrate8/2(In2), Substrate7/2(In2)

== system MIL_ASW/Application_Software_SHAW/ASW_GearPressureControl/Fork 1 ==
  ForkDirReq : Inport
  ForkSyncPha : Inport  Port=2
  ForkDeltaSpdReq : Inport  Port=3
  ForkPosnReq : Inport  Port=4
  ForkDeltaSpdAct : Inport  Port=5
  ForkPosnVal : Inport  Port=6
  Enable : EnablePort  StatesWhenEnabling=reset
  Abs : Abs  OutDataTypeStr=uint16
  Abs2 : Abs  OutDataTypeStr=uint16
  Add4 : Sum  Inputs=+-  OutDataTypeStr=int16
  Add6 : Sum  Inputs=+-  OutDataTypeStr=int16
  Compare To Constant : simulink/Logic and Bit Operations/Compare To Constant  relop===  const=2  OutDataTypeStr=boolean
  Compare To Constant1 : simulink/Logic and Bit Operations/Compare To Constant  relop===  const=1  OutDataTypeStr=boolean
  Compare To Constant2 : simulink/Logic and Bit Operations/Compare To Constant  relop===  const=3  OutDataTypeStr=boolean
  Compare To Constant3 : simulink/Logic and Bit Operations/Compare To Constant  relop===  const=2  OutDataTypeStr=boolean
  Compare To Constant4 : simulink/Logic and Bit Operations/Compare To Constant  relop===  const=4  OutDataTypeStr=boolean
  Constant : Constant  Value=150  OutDataTypeStr=uint16
  Gain : Gain  Gain=5  OutDataTypeStr=uint16
  Gain1 : Gain  OutDataTypeStr=uint16
  Logical Operator : Logic  Operator=OR  AllPortsSameDT=off  OutDataTypeStr=boolean
  Logical Operator1 : Logic  Operator=OR  AllPortsSameDT=off  OutDataTypeStr=boolean
  Saturation : Saturate  UpperLimit=300  LowerLimit=0  OutDataTypeStr=uint16
  Switch : Switch  Criteria=u2 > Threshold
  Switch1 : Switch  Criteria=u2 > Threshold
  Switch2 : Switch  Criteria=u2 > Threshold
  Terminator : Terminator
  ForkPReq : Outport  VectorParamsAs1DForOutWhenUnconnected=off
  wires:
  ForkPosnReq/1 -> Switch1/1, Switch2/1
  ForkDeltaSpdReq/1 -> Add6/1
  ForkDeltaSpdAct/1 -> Add6/2
  Add6/1 -> Abs2/1
  Add4/1 -> Abs/1
  Abs2/1 -> Gain1/1
  Compare To Constant/1 -> Switch/2
  ForkSyncPha/1 -> Compare To Constant/1
  Constant/1 -> Switch/1
  Gain/1 -> Switch/3
  ForkDirReq/1 -> Compare To Constant3/1, Compare To Constant1/1, Compare To Constant4/1, Compare To Constant2/1
  Compare To Constant1/1 -> Logical Operator/1
  Compare To Constant3/1 -> Logical Operator/2
  Compare To Constant2/1 -> Logical Operator1/1
  Compare To Constant4/1 -> Logical Operator1/2
  Logical Operator/1 -> Switch1/2
  ForkPosnVal/1 -> Switch2/3, Switch1/3
  Logical Operator1/1 -> Switch2/2
  Switch1/1 -> Add4/1
  Switch2/1 -> Add4/2
  Switch/1 -> Saturation/1
  Saturation/1 -> ForkPReq/1
  Gain1/1 -> Terminator/1
  Abs/1 -> Gain/1

== system MIL_ASW/Application_Software_SHAW/ASW_GearPressureControl/Fork 2 ==
  ForkDirReq : Inport
  ForkSyncPha : Inport  Port=2
  ForkDeltaSpdReq : Inport  Port=3
  ForkPosnReq : Inport  Port=4
  ForkDeltaSpdAct : Inport  Port=5
  ForkPosnVal : Inport  Port=6
  Enable : EnablePort  StatesWhenEnabling=reset
  Abs : Abs  OutDataTypeStr=uint16
  Abs2 : Abs  OutDataTypeStr=uint16
  Add4 : Sum  Inputs=+-  OutDataTypeStr=int16
  Add6 : Sum  Inputs=+-  OutDataTypeStr=int16
  Compare To Constant : simulink/Logic and Bit Operations/Compare To Constant  relop===  const=2  OutDataTypeStr=boolean
  Compare To Constant1 : simulink/Logic and Bit Operations/Compare To Constant  relop===  const=1  OutDataTypeStr=boolean
  Compare To Constant2 : simulink/Logic and Bit Operations/Compare To Constant  relop===  const=3  OutDataTypeStr=boolean
  Compare To Constant3 : simulink/Logic and Bit Operations/Compare To Constant  relop===  const=2  OutDataTypeStr=boolean
  Compare To Constant4 : simulink/Logic and Bit Operations/Compare To Constant  relop===  const=4  OutDataTypeStr=boolean
  Constant : Constant  Value=150  OutDataTypeStr=uint16
  Gain : Gain  Gain=5  OutDataTypeStr=uint16
  Gain1 : Gain  OutDataTypeStr=uint16
  Logical Operator : Logic  Operator=OR  AllPortsSameDT=off  OutDataTypeStr=boolean
  Logical Operator1 : Logic  Operator=OR  AllPortsSameDT=off  OutDataTypeStr=boolean
  Saturation : Saturate  UpperLimit=300  LowerLimit=0  OutDataTypeStr=uint16
  Switch : Switch  Criteria=u2 > Threshold
  Switch1 : Switch  Criteria=u2 > Threshold
  Switch2 : Switch  Criteria=u2 > Threshold
  Terminator : Terminator
  ForkPReq : Outport  VectorParamsAs1DForOutWhenUnconnected=off
  wires:
  Abs/1 -> Gain/1
  Gain1/1 -> Terminator/1
  Saturation/1 -> ForkPReq/1
  Switch/1 -> Saturation/1
  Switch2/1 -> Add4/2
  Switch1/1 -> Add4/1
  Logical Operator1/1 -> Switch2/2
  ForkPosnVal/1 -> Switch1/3, Switch2/3
  Logical Operator/1 -> Switch1/2
  Compare To Constant4/1 -> Logical Operator1/2
  Compare To Constant2/1 -> Logical Operator1/1
  Compare To Constant3/1 -> Logical Operator/2
  Compare To Constant1/1 -> Logical Operator/1
  ForkDirReq/1 -> Compare To Constant2/1, Compare To Constant4/1, Compare To Constant1/1, Compare To Constant3/1
  Gain/1 -> Switch/3
  Constant/1 -> Switch/1
  ForkSyncPha/1 -> Compare To Constant/1
  Compare To Constant/1 -> Switch/2
  Abs2/1 -> Gain1/1
  Add4/1 -> Abs/1
  Add6/1 -> Abs2/1
  ForkDeltaSpdAct/1 -> Add6/2
  ForkDeltaSpdReq/1 -> Add6/1
  ForkPosnReq/1 -> Switch2/1, Switch1/1
